simulink model "railway02"  (Simulink 6.5)
settings: Solver=FixedStepDiscrete  StartTime=0.0  StopTime=inf  FixedStep=0.01  RelTol=1e-3
libraries: simulink x1
settings Model: Creator=sja  LastModifiedBy=haf  ExtModeAutoUpdateStatusClock=off
settings DebuggingCC: MultiTaskDSMMsg=warning  MultiTaskCondExecSysMsg=none  StrictBusMsg=None
settings RTWCC: IncludeERTFirstTime=on

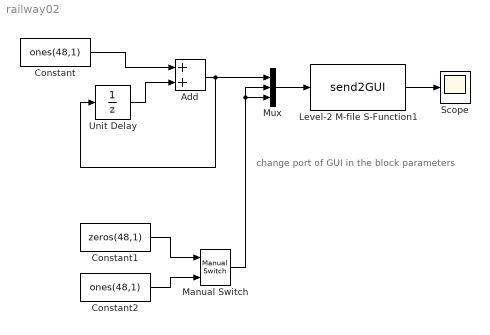
== system railway02 ==
  note: change port of
      | GUI in the block
      | parameters
  Add : Sum  OutScaling=2^-10
  Constant : Constant  Value=ones(48,1)  OutDataType=sfix(16)  ConRadixGroup=Use specified scaling  OutScaling=2^0  SampleTime=inf  FramePeriod=inf
  Constant1 : Constant  Value=zeros(48,1)  OutDataType=sfix(16)  ConRadixGroup=Use specified scaling  OutScaling=2^0  SampleTime=inf  FramePeriod=inf
  Constant2 : Constant  Value=ones(48,1)  OutDataType=sfix(16)  ConRadixGroup=Use specified scaling  OutScaling=2^0  SampleTime=inf  FramePeriod=inf
  Level-2 M-file S-Function1 : M-S-Function  FunctionName=send2GUI  Parameters=port,dimensions,sampletime  mask{port=12345, dimensions=0, sampletime=-1}
      mask prompts: port "TCP Port for GUI server"; dimensions "Output Port Dimensions"
      mask help: Interface Block to pass data between the model and a graphical user interface accessed via TCP/IP.
      mask Display:
      | fprintf('GUI INTERFACE\n\n')
      | fprintf(['Port: ' num2str(port)])
  Manual Switch : simulink/Signal Routing/Manual Switch  SystemSampleTime=-1  sw=1  action=0
  Mux : Mux  Inputs=3
  Scope : Scope
      settings: YMin=0.95  YMax=1.05
  Unit Delay : UnitDelay
  wires:
  Level-2 M-file S-Function1/1 -> Scope/1
  Add/1 -> Unit Delay/1, Mux/1
  Constant/1 -> Add/1
  Unit Delay/1 -> Add/2
  Mux/1 -> Level-2 M-file S-Function1/1
  Manual Switch/1 -> Mux/2, Mux/3
  Constant1/1 -> Manual Switch/1
  Constant2/1 -> Manual Switch/2
